simulink model "appint_ros_example"  (Simulink 9.2)
settings: Solver=FixedStepDiscrete  StartTime=0.0  StopTime=inf  FixedStep=1e-3  RelTol=1e-3
values from neighbouring files (symbols this model uses):
  g_base = [0;0;-9.81]    [appint_ros_example_open.m]
  pkin = 0.4    [appint_ros_example_open.m]
  q_t0 = zeros(2,1)    [appint_ros_example_open.m]
  qD_t0 = zeros(2,1)    [appint_ros_example_open.m]
undefined symbols (not defined in the file or in its folder): DiscIntNeverNeededParam
undefined symbols (not defined in the file): DynPar1
settings Model: LogicAnalyzerSignalOrdering=12c0b665-86dc-437a-a1c1-0f1ba1b57c4d  Creator=moritz  LastModifiedBy=schappler  SimulationMode=external  ExtModeTrigDuration=10000  ExtModeArchiveMode=auto  ExtModeArchiveFileName=measurement_data  ExtModeArchiveDirName=./results
settings DataIOCC: LimitDataPoints=off  SaveFormat=Dataset  SignalLoggingSaveFormat=Dataset  SaveOutput=off  SignalLogging=off  SaveTime=off
settings OptimizationCC: BlockReduction=off  ConditionallyExecuteInputs=off  OptimizeBlockIOStorage=off  BufferReuse=off  GlobalBufferReuse=off  ExpressionFolding=off  LocalBlockOutputs=off  LifeSpan=auto  OptimizeDataStoreBuffers=off  BusAssignmentInplaceUpdate=off
settings DebuggingCC: UnderspecifiedInitializationDetection=Simplified  MergeDetectMultiDrivingBlocksExec=error  FcnCallInpInsideContextMsg=error  StateNameClashWarn=none  SFUnexpectedBacktrackingDiag=error  SFNoUnconditionalDefaultTransitionDiag=error  SFExecutionAtInitializationDiag=warning
settings HardwareCC: ProdBitPerPointer=64  ProdBitPerSizeT=64  ProdBitPerPtrDiffT=64  ProdLargestAtomicFloat=Float  ProdIntDivRoundTo=Zero  ProdEndianess=LittleEndian  ProdWordSize=64  ProdHWDeviceType=Intel->x86-64 (Windows64)
settings ModelReferenceCC: PropagateSignalLabelsOutOfModel=on
settings RTWCC: SystemTargetFile=etherlab.tlc  TemplateMakefile=etherlab_hrt.tmf  Description=EtherLab PREEMT_RT Real-Time Target
settings CodeAppCC: StateflowObjectComments=off
settings STFCustomTargetCC: TargetLangStandard=C99 (ISO)  ModelReferenceCompliant=off  SystemTargetFile=etherlab.tlc
settings GRTTargetCC: TargetLangStandard=C99 (ISO)  ModelReferenceCompliant=off  ParMdlRefBuildCompliant=off  CompOptLevelCompliant=off  ConcurrentExecutionCompliant=off  GeneratePreprocessorConditionals=Use local settings  MatFileLogging=off  CPPClassGenCompliant=off  UseToolchainInfoCompliant=off  ExtMode=on  ExtModeStaticAlloc=on  ExtModeStaticAllocSize=10000000  ExtModeMexArgs='10.144.130.83' 0 17725  RTWCAPISignals=on  RTWCAPIParams=on
settings CustomProperty: DataType=int32  Value=2
settings ConfigComp: CovMetricSettings=dwe  CovHtmlReporting=off  CovSaveCumulativeToWorkspaceVar=off  CovSaveSingleToWorkspaceVar=off  CovExternalEMLEnable=on

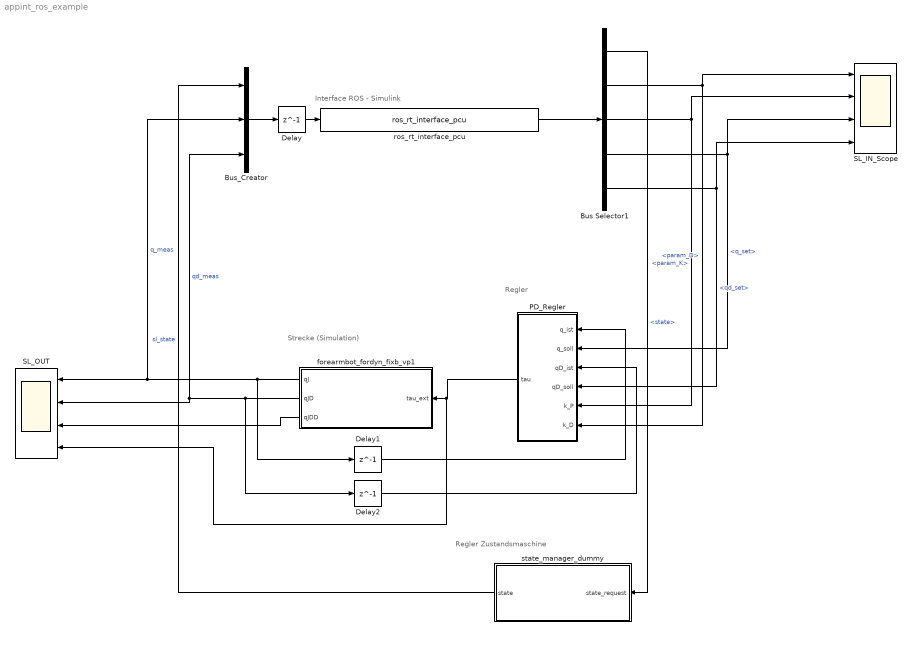
== system appint_ros_example ==
  note: Regler
  note: Interface ROS - Simulink
  note: Strecke (Simulation)
  note: Regler Zustandsmaschine
  Bus Selector1 : BusSelector  OutputSignals=state,param_D,param_K,q_set,qd_set
  Bus_Creator : BusCreator  Inputs=3
  Delay : Delay  DelayLength=1
  Delay1 : Delay  DelayLength=1  InitialCondition=0
  Delay2 : Delay  DelayLength=1  InitialCondition=0
  PD_Regler : Subsystem
  SL_IN_Scope : Scope  NumInputPorts=4
  SL_OUT : Scope  NumInputPorts=4
  forearmbot_fordyn_fixb_vp1 : Subsystem  mask{q_t0=q_t0, qD_t0=qD_t0, g_base=g_base, pkin=pkin, DynPar1=DynPar1}
      mask prompts: q_t0 "q0 (initial pose)"; qD_t0 "qD0 (initial velocity)"; pkin "Kinematik-Parameter"; DynPar1 "Dynamik-Parameter (Parametersatz 1)"
      mask init:
      | NQJ=2;
  ros_rt_interface_pcu : S-Function  FunctionName=ros_rt_interface_pcu  SFunctionDeploymentMode=off  EnableBusSupport=off  mask(Legacy Function){SFunctionSpec=void SL_io_func(SL_OUT_type u1[1], SL_IN_type y1[1]), ShowSpec=on}
      mask prompts: ShowSpec "Display function specification"
      mask help:
      | This block allows you to call the legacy functions specified by the following Legacy Code Tool definition:
      | def.SFunctionName = 'ros_rt_interface_pcu';
      | def.OutputFcnSpec = 'void SL_io_func(SL_OUT_type u1[1], SL_IN_type y1[1])';
      | def.StartFcnSpec = 'void SL_start_func()';
      | def.TerminateFcnSpec = 'void SL_terminate_func()';
      | def.HeaderFiles = {'SL_func.h'};
      | def.SourceFiles = {'../ros_rt_interface/ros_rt_core/SL_func_dummy.cpp'};
      | def.TargetLibFiles = {'libros_sl_interface.so'};
      | def.IncPaths = {'../ros_rt_interface/ros_rt_core'};
      mask Help: <p>This block was generated automatically by the Legacy Code Tool. For detailed help on this tool, call<a href="matlab:legacy_code('help')"> legacy_code('help')</a>.</p>
      mask Callback ShowSpec:
      | if strcmp(get_param(gcbh, 'ShowSpec'), 'on')
      |   set_param(gcbh, 'MaskDisplay', sprintf('fprintf(''%s'');', get_param(gcbh, 'SFunctionSpec')));
      | else
      |   set_param(gcbh, 'MaskDisplay', sprintf('fprintf(''%s'');', get_param(gcbh, 'FunctionName')));
      | end
      mask Display: fprintf('void SL_io_func(SL_OUT_type u1[1], SL_IN_type y1[1])');
  state_manager_dummy : Subsystem
  wires:
  Delay/1 -> ros_rt_interface_pcu/1
  Bus_Creator/1 -> Delay/1
  ros_rt_interface_pcu/1 -> Bus Selector1/1
  PD_Regler/1(tau) -> SL_OUT/4, forearmbot_fordyn_fixb_vp1/1("tau_ext ")
  forearmbot_fordyn_fixb_vp1/1(qJ) -> Delay1/1, SL_OUT/1, Bus_Creator/2  "q_meas"
  forearmbot_fordyn_fixb_vp1/2(qJD) -> Delay2/1, Bus_Creator/3, SL_OUT/2  "qd_meas"
  Delay1/1 -> PD_Regler/1(q_ist)
  Delay2/1 -> PD_Regler/3(qD_ist)
  Bus Selector1/4 -> SL_IN_Scope/3, PD_Regler/2(q_soll)  "<q_set>"
  Bus Selector1/5 -> SL_IN_Scope/4, PD_Regler/4(qD_soll)  "<qd_set>"
  Bus Selector1/2 -> SL_IN_Scope/1, PD_Regler/6(k_D)  "<param_D>"
  Bus Selector1/3 -> SL_IN_Scope/2, PD_Regler/5(k_P)  "<param_K>"
  Bus Selector1/1 -> state_manager_dummy/1(state_request)  "<state>"
  state_manager_dummy/1(state) -> Bus_Creator/1  "sl_state"
  forearmbot_fordyn_fixb_vp1/3(qJDD) -> SL_OUT/3

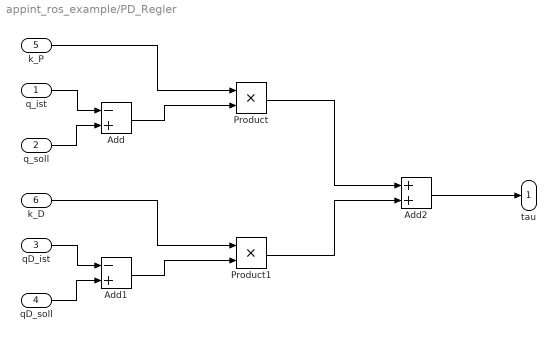
== system appint_ros_example/PD_Regler ==
  q_ist : Inport  PortDimensions=[2 1]
  q_soll : Inport  Port=2  PortDimensions=[2 1]
  qD_ist : Inport  Port=3  PortDimensions=[2 1]
  qD_soll : Inport  Port=4  PortDimensions=[2 1]
  k_P : Inport  Port=5  PortDimensions=[2 1]
  k_D : Inport  Port=6  PortDimensions=[2 1]
  Add : Sum  Inputs=-+
  Add1 : Sum  Inputs=-+
  Add2 : Sum
  Product : Product
  Product1 : Product
  tau : Outport
  wires:
  k_P/1 -> Product/1
  q_soll/1 -> Add/2
  q_ist/1 -> Add/1
  k_D/1 -> Product1/1
  Add1/1 -> Product1/2
  qD_soll/1 -> Add1/2
  qD_ist/1 -> Add1/1
  Product/1 -> Add2/1
  Product1/1 -> Add2/2
  Add2/1 -> tau/1
  Add/1 -> Product/2

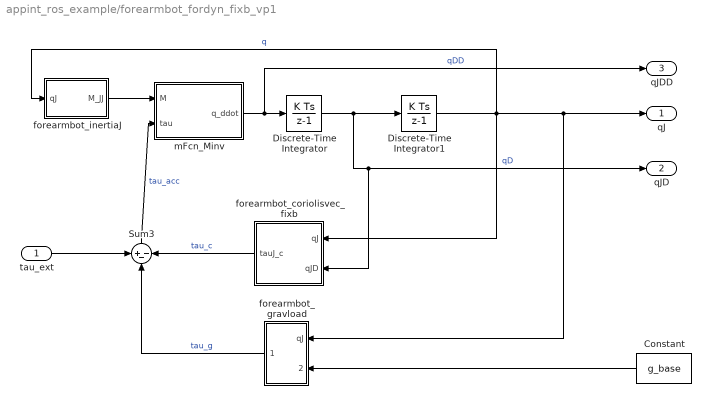
== system appint_ros_example/forearmbot_fordyn_fixb_vp1 ==
  "tau_ext " : Inport  PortDimensions=NQJ
  Constant : Constant  Value=g_base
  Discrete-Time Integrator : DiscreteIntegrator  InitialCondition=qD_t0  SampleTime=-1  ICPrevOutput=DiscIntNeverNeededParam  ICPrevScaledInput=DiscIntNeverNeededParam
  Discrete-Time Integrator1 : DiscreteIntegrator  InitialCondition=q_t0  SampleTime=-1  ICPrevOutput=DiscIntNeverNeededParam  ICPrevScaledInput=DiscIntNeverNeededParam
  Sum3 : Sum  Inputs=+--
  forearmbot_coriolisvec_fixb : Subsystem  mask{pkin=pkin, DynPar1=DynPar1}
      mask prompts: pkin "Kinematik-Parameter"; DynPar1 "Dynamik-Parameter (Parametersatz 1)"
      mask init:
      | NQJ=2;
      | m = DynPar1.m;
      | r_S = DynPar1.r_S;
      | I_S = DynPar1.I_S;
  forearmbot_gravload : Subsystem  mask{pkin=pkin, DynPar1=DynPar1}
      mask prompts: pkin "Kinematik-Parameter"; DynPar1 "Dynamik-Parameter (Parametersatz 1)"
      mask init:
      | NQJ=2;
      | m = DynPar1.m;
      | r_S = DynPar1.r_S;
      | I_S = DynPar1.I_S;
  forearmbot_inertiaJ : Subsystem  mask{pkin=pkin, DynPar1=DynPar1}
      mask prompts: pkin "Kinematik-Parameter"; DynPar1 "Dynamik-Parameter (Parametersatz 1)"
      mask init:
      | NQJ=2;
      | m = DynPar1.m;
      | r_S = DynPar1.r_S;
      | I_S = DynPar1.I_S;
  mFcn_Minv : MATLAB Function  TreatAsAtomicUnit=on
  qJ : Outport  PortDimensions=NQJ
  qJD : Outport  Port=2  PortDimensions=NQJ
  qJDD : Outport  Port=3  PortDimensions=NQJ
  wires:
  forearmbot_gravload/1(tau_g) -> Sum3/2  "tau_g"
  Discrete-Time Integrator1/1 -> forearmbot_coriolisvec_fixb/1(qJ), forearmbot_inertiaJ/1(qJ), forearmbot_gravload/1(qJ), qJ/1  "q"
  mFcn_Minv/1(q_ddot) -> Discrete-Time Integrator/1, qJDD/1  "qDD"
  forearmbot_coriolisvec_fixb/1(tauJ_c) -> Sum3/3  "tau_c"
  "tau_ext "/1 -> Sum3/1
  Discrete-Time Integrator/1 -> Discrete-Time Integrator1/1, forearmbot_coriolisvec_fixb/2(qJD), qJD/1  "qD"
  Sum3/1 -> mFcn_Minv/2(tau)  "tau_acc"
  forearmbot_inertiaJ/1(M_JJ) -> mFcn_Minv/1(M)
  Constant/1 -> forearmbot_gravload/2(g_base)

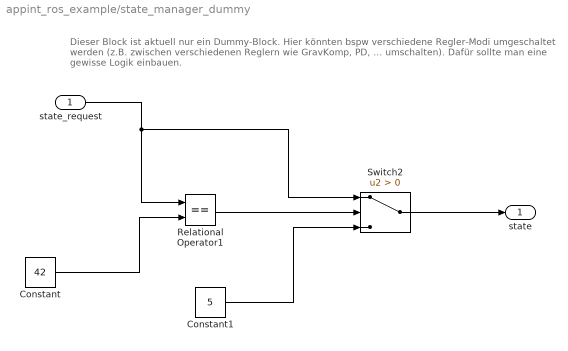
== system appint_ros_example/state_manager_dummy ==
  note: Dieser Block ist aktuell nur ein Dummy-Block. Hier könnten bspw verschiedene Regler-Modi umgeschaltet werden
      | (z.B. zwischen verschiedenen Reglern wie GravKomp, PD, ... umschalten). Dafür sollte man eine gewisse Logik einbauen.
  state_request : Inport  OutDataTypeStr=uint8
  Constant : Constant  Value=42  OutDataTypeStr=uint8
  Constant1 : Constant  Value=5  OutDataTypeStr=uint8
  Relational Operator1 : RelationalOperator  Operator===  OutDataTypeStr=boolean  RndMeth=Simplest
  Switch2 : Switch  Criteria=u2 > Threshold
  state : Outport  OutDataTypeStr=uint8
  wires:
  Constant1/1 -> Switch2/3
  state_request/1 -> Switch2/1, Relational Operator1/1
  Switch2/1 -> state/1
  Constant/1 -> Relational Operator1/2
  Relational Operator1/1 -> Switch2/2

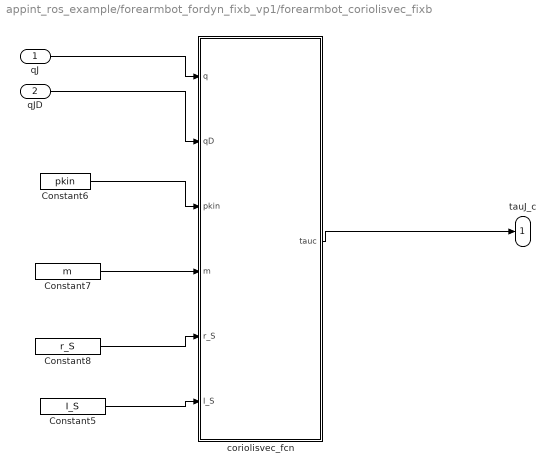
== system appint_ros_example/forearmbot_fordyn_fixb_vp1/forearmbot_coriolisvec_fixb ==
  qJ : Inport  PortDimensions=NQJ
  qJD : Inport  Port=2  PortDimensions=NQJ
  Constant5 : Constant  Value=I_S
  Constant6 : Constant  Value=pkin
  Constant7 : Constant  Value=m
  Constant8 : Constant  Value=r_S
  coriolisvec_fcn : MATLAB Function  TreatAsAtomicUnit=on
  tauJ_c : Outport  PortDimensions=NQJ
  wires:
  Constant5/1 -> coriolisvec_fcn/6(I_S)
  Constant8/1 -> coriolisvec_fcn/5(r_S)
  Constant7/1 -> coriolisvec_fcn/4(m)
  qJ/1 -> coriolisvec_fcn/1(q)
  qJD/1 -> coriolisvec_fcn/2(qD)
  Constant6/1 -> coriolisvec_fcn/3(pkin)
  coriolisvec_fcn/1(tauc) -> tauJ_c/1

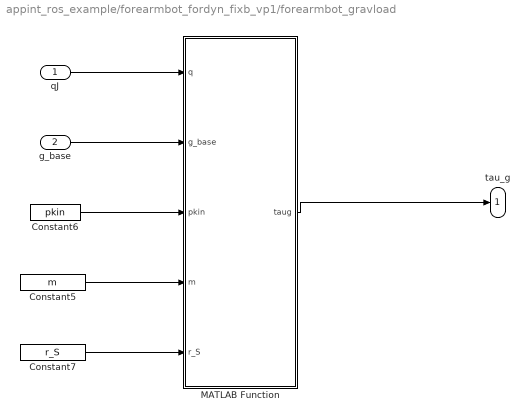
== system appint_ros_example/forearmbot_fordyn_fixb_vp1/forearmbot_gravload ==
  qJ : Inport  PortDimensions=NQJ
  g_base : Inport  Port=2  PortDimensions=3
  Constant5 : Constant  Value=m
  Constant6 : Constant  Value=pkin
  Constant7 : Constant  Value=r_S
  MATLAB Function : MATLAB Function  TreatAsAtomicUnit=on
  tau_g : Outport  PortDimensions=NQJ
  wires:
  Constant7/1 -> MATLAB Function/5(r_S)
  Constant5/1 -> MATLAB Function/4(m)
  qJ/1 -> MATLAB Function/1(q)
  g_base/1 -> MATLAB Function/2(g_base)
  Constant6/1 -> MATLAB Function/3(pkin)
  MATLAB Function/1(taug) -> tau_g/1

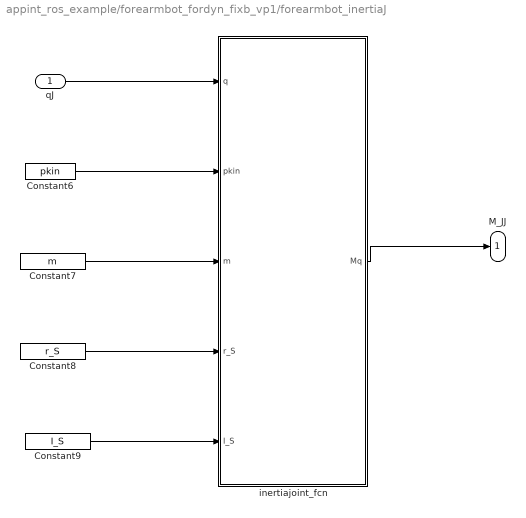
== system appint_ros_example/forearmbot_fordyn_fixb_vp1/forearmbot_inertiaJ ==
  qJ : Inport  PortDimensions=NQJ
  Constant6 : Constant  Value=pkin
  Constant7 : Constant  Value=m
  Constant8 : Constant  Value=r_S
  Constant9 : Constant  Value=I_S
  inertiajoint_fcn : MATLAB Function  TreatAsAtomicUnit=on
  M_JJ : Outport  PortDimensions=[NQJ NQJ]
  wires:
  Constant9/1 -> inertiajoint_fcn/5(I_S)
  Constant8/1 -> inertiajoint_fcn/4(r_S)
  Constant7/1 -> inertiajoint_fcn/3(m)
  qJ/1 -> inertiajoint_fcn/1(q)
  Constant6/1 -> inertiajoint_fcn/2(pkin)
  inertiajoint_fcn/1(Mq) -> M_JJ/1

== matlab function forearmbot_fordyn_fixb_vp1/forearmbot_gravload/MATLAB Function ==
  data: q input double; taug output double; g_base input double; pkin input double; m input double; r_S input double
function taug = gravload(q, g_base, pkin, m, r_S)
%#codegen
taug = forearmbot_gravloadJ_floatb_twist_slag_vp1(q, g_base, pkin, m, r_S);

end

function taug = forearmbot_gravloadJ_floatb_twist_slag_vp1(qJ, g, ...
  pkin, m, rSges)

%% Symbolic Calculation
% From gravload_joint_floatb_twist_par1_matlab.m
% OptimizationMode: 2
% StartTime: 2020-03-31 10:54:15
% EndTime: 2020-03-31 10:54:15
% DurationCPUTime: 0.11s
% Computational Cost: add. (1->1), mult. (6->5), div. (0->0), fcn. (2->2), ass. (0->1)
t1 = [(m(2) * sin(qJ(1)) * rSges(2,1) + m(3) * cos(qJ(1)) * pkin(1)) * g(3), 0];
taug = t1(:);

end

== matlab function forearmbot_fordyn_fixb_vp1/forearmbot_coriolisvec_fixb/coriolisvec_fcn ==
  data: q input double; tauc output double; qD input double; pkin input double; m input double; r_S input double; I_S input double
function tauc = coriolis(q, qD, pkin, m, r_S, I_S)
%#codegen
tauc = forearmbot_coriolisvecJ_fixb_slag_vp1(q, qD, pkin, m, r_S, I_S);

end

function tauc = forearmbot_coriolisvecJ_fixb_slag_vp1(qJ, qJD, ...
  pkin, m, rSges, Icges)

%% Symbolic Calculation
% From coriolisvec_joint_fixb_par1_matlab.m
% OptimizationMode: 2
% StartTime: 2020-03-31 10:54:15
% EndTime: 2020-03-31 10:54:16
% DurationCPUTime: 0.75s
% Computational Cost: add. (228->55), mult. (1048->101), div. (0->0), fcn. (610->4), ass. (0->47)
t27 = sin(qJ(1));
t26 = sin(qJ(2));
t28 = cos(qJ(2));
t46 = Icges(3,1) - Icges(3,2);
t65 = t46 * t28 * t26;
t15 = t27 * t65;
t22 = t26 ^ 2;
t24 = t28 ^ 2;
t39 = Icges(3,1) * t24 + Icges(3,2) * t22;
t64 = 2 * qJD(2);
t36 = -Icges(3,3) + t39;
t66 = t27 * t36;
t23 = t27 ^ 2;
t29 = cos(qJ(1));
t25 = t29 ^ 2;
t16 = Icges(3,3) * t25 + t39 * t23;
t62 = t27 / 0.2e1;
t61 = -t29 / 0.2e1;
t60 = t29 / 0.2e1;
t11 = t29 * t66;
t59 = t11 * t27;
t58 = t11 * t29;
t14 = t29 * t65;
t57 = t14 * t29;
t56 = t15 * t27;
t55 = t16 * t27;
t17 = t23 * Icges(3,3) + t25 * t39;
t54 = t17 * t29;
t47 = qJD(1) * t29;
t13 = t14 * qJD(1);
t33 = t46 * (t22 - t24);
t32 = qJD(2) * t33;
t4 = t27 * t32 - t13;
t37 = qJD(1) * t65;
t5 = t27 * t37 + t29 * t32;
t40 = -t5 * t27 + t4 * t29;
t38 = qJD(2) * t65;
t12 = t27 * t14;
t35 = (t16 * t29 - t59) * qJD(2);
t34 = (-t17 * t27 + t58) * qJD(2);
t10 = t33 * t29;
t9 = t33 * t27;
t8 = -t16 + t17;
t3 = -t12 * t64 + (-t23 + t25) * qJD(1) * t36;
t2 = -t15 * qJD(1) + t35;
t1 = -t13 + t34;
t6 = [(t2 * t62 - t13 * t61 + t1 * t60 + ((-t27 * t8 - t55 + t58) * t61 + (t29 * t8 - t54 + t59) * t62) * qJD(2) + (0.3e1 / 0.2e1 * t56 + t57 + 0.2e1 * t65) * qJD(1) + t40) * qJD(2); qJD(1) * ((t56 + t57) * qJD(1) + t40) / 0.2e1 - (t5 * qJD(1) + (-0.2e1 * t27 * (-t25 * t38 - t47 * t66) + t3 * t29 + (-t54 - t59) * qJD(1)) * t64) * t27 / 0.2e1 + (t4 * qJD(1) + (0.2e1 * t29 * (qJD(1) * t11 - t23 * t38) - t3 * t27 + (-t55 - t58) * qJD(1)) * t64) * t60 - (t1 + t34) * t47 / 0.2e1 + ((t9 * qJD(1) + (t12 * t27 - t23 * t14) * t64) * t61 + (t10 * qJD(1) + (-t12 * t29 + t15 * t25) * t64) * t62) * qJD(2) - (0.2e1 * t37 + (t2 + t35) * t27 + (-t10 * t27 + t9 * t29) * qJD(2)) * qJD(1) / 0.2e1;];
tauc = t6(:);
end

== matlab function forearmbot_fordyn_fixb_vp1/forearmbot_inertiaJ/inertiajoint_fcn ==
  data: q input double; Mq output double; pkin input double; m input double; r_S input double; I_S input double
function Mq = inertia(q, pkin, m, r_S, I_S)
%#codegen
Mq = forearmbot_inertiaJ_slag_vp1(q, pkin, m, r_S, I_S);

end

function Mq = forearmbot_inertiaJ_slag_vp1(qJ, ...
  pkin, m, rSges, Icges)

%% Symbolic Calculation
% From inertia_joint_joint_floatb_twist_par1_matlab.m
% OptimizationMode: 2
% StartTime: 2020-03-31 10:54:15
% EndTime: 2020-03-31 10:54:15
% DurationCPUTime: 0.17s
% Computational Cost: add. (20->7), mult. (84->15), div. (0->0), fcn. (52->4), ass. (0->7)
t7 = sin(qJ(1));
t3 = t7 ^ 2;
t9 = cos(qJ(1));
t5 = t9 ^ 2;
t8 = cos(qJ(2));
t6 = sin(qJ(2));
t1 = [t6 ^ 2 * Icges(3,1) + t8 ^ 2 * Icges(3,2) + Icges(2,3) + (m(2) * rSges(2,1) ^ 2 + m(3) * pkin(1) ^ 2) * (t3 + t5); 0; (t5 ^ 2 + (0.2e1 * t5 + t3) * t3) * Icges(3,3);];
%% Postprocessing: Reshape Output
% From vec2symmat_2_matlab.m
res = [t1(1), t1(2); t1(2), t1(3);];
Mq = res;

end

== matlab function forearmbot_fordyn_fixb_vp1/mFcn_Minv ==
  data: M input double; q_ddot output double; tau input double
function q_ddot = fcn(M,tau)
%#codegen
q_ddot=M\tau;
